simulink model "PhysicalLeanBroth"  (R2026a)
settings: Solver=VariableStepAuto  StopTime=14400
undefined symbols (not defined in the file): Fault_T_Kettle1, Fault_T_Kettle2, Fault_T_Pack, Fault_T_Prep, Fault_T_QC, LB_PackRate_bph, LB_QCRate_bph, LB_Resupply_bph, Recipe_Block_s, Recipe_Count, Resupply_Cutoff_T, Transport_Latency_s, Transport_Rate_bph
(part 1 of 2)
settings Model: DataDictionary=PhysicalLeanBrothData.sldd  Creator=sarah  LastModifiedBy=sarah

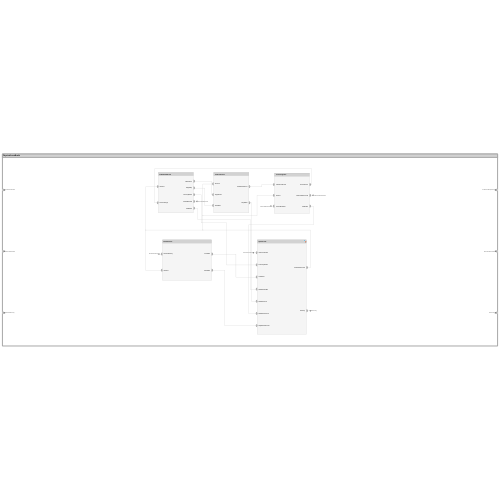
[thumbnail: Simulink's stored preview of the top-level diagram]
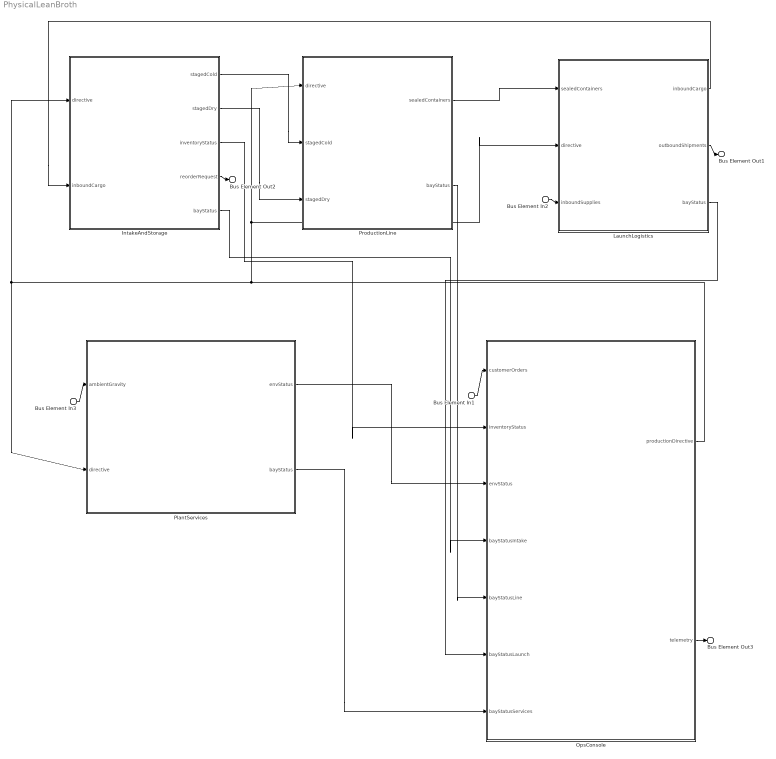
== system PhysicalLeanBroth ==
  Bus Element In1 : Inport  PortName=CustomerOrders
  Bus Element In2 : Inport  Port=2  PortName=InboundSupplies
  Bus Element In3 : Inport  Port=3  PortName=AmbientGravity
  IntakeAndStorage : Subsystem
      settings: PortSchema="{\"entries\":[{\"content\":{\"headerSize\":26,\"margin\":15,\"minimumSpacing\":25,\"sides\":[{\"content\":{\"connectorIds\":[\"In1\",\"In2\"]},\"type\":\"ConnectorPlacement.EquallySpacedRectSide\",\"uuid\":\"3a94c7fc-0b9e-4df5-a2de-1d2483378dcb\"},{\"content\":{\"connectorIds\":[\"Out1\",\"Out2\",\"Out3\",\"Out4\",\"Out5\"],\"side\":\"RIGHT\"},\"type\":\"ConnectorPlacement.EquallySpacedRectSide\",\"uuid\":\"607e1f04-41cc-4c9a-b401-96cdf33819d0\"},{\"content\":{\"side\":\"TOP\"},\"type\":\"ConnectorPlacement.EquallySpacedRectSide\",\"uuid\":\"2ee07fc7-54c6-4cee-9888-3f37ad01f332\"}]},\"type\":\"ConnectorPlacement.EquallySpacedConnector\",\"uuid\":\"f91f3af9-eaeb-4625-ae6e-5ceb7fb8b64c\"}],\"packageUris\":[\"http://schema.mathworks.com/mf0/Connector/R2020b\"],\"version\":\"1.0\"}"
  LaunchLogistics : Subsystem
      settings: PortSchema="{\"entries\":[{\"content\":{\"headerSize\":26,\"margin\":15,\"minimumSpacing\":25,\"sides\":[{\"content\":{\"connectorIds\":[\"In1\",\"In2\",\"In3\"]},\"type\":\"ConnectorPlacement.EquallySpacedRectSide\",\"uuid\":\"3a94c7fc-0b9e-4df5-a2de-1d2483378dcb\"},{\"content\":{\"connectorIds\":[\"Out1\",\"Out2\",\"Out3\"],\"side\":\"RIGHT\"},\"type\":\"ConnectorPlacement.EquallySpacedRectSide\",\"uuid\":\"607e1f04-41cc-4c9a-b401-96cdf33819d0\"},{\"content\":{\"side\":\"TOP\"},\"type\":\"ConnectorPlacement.EquallySpacedRectSide\",\"uuid\":\"2ee07fc7-54c6-4cee-9888-3f37ad01f332\"}]},\"type\":\"ConnectorPlacement.EquallySpacedConnector\",\"uuid\":\"f91f3af9-eaeb-4625-ae6e-5ceb7fb8b64c\"}],\"packageUris\":[\"http://schema.mathworks.com/mf0/Connector/R2020b\"],\"version\":\"1.0\"}"
  OpsConsole : Subsystem
      settings: PortSchema="{\"entries\":[{\"content\":{\"headerSize\":26,\"margin\":15,\"minimumSpacing\":25,\"sides\":[{\"content\":{\"connectorIds\":[\"In1\",\"In2\",\"In3\",\"In4\",\"In5\",\"In6\",\"In7\"]},\"type\":\"ConnectorPlacement.EquallySpacedRectSide\",\"uuid\":\"f830f98a-8e8b-4468-adf4-d6eab644987f\"},{\"content\":{\"connectorIds\":[\"Out1\",\"Out2\"],\"side\":\"RIGHT\"},\"type\":\"ConnectorPlacement.EquallySpacedRectSide\",\"uuid\":\"7e0d0116-b3ba-4668-b638-30d0f54ba087\"},{\"content\":{\"side\":\"TOP\"},\"type\":\"ConnectorPlacement.EquallySpacedRectSide\",\"uuid\":\"7b4146d3-46d2-45ca-8c34-b106f0d8cedd\"}]},\"type\":\"ConnectorPlacement.EquallySpacedConnector\",\"uuid\":\"3d911b2d-a78f-42ea-b869-5e09982d9f54\"}],\"packageUris\":[\"http://schema.mathworks.com/mf0/Connector/R2020b\"],\"version\":\"1.0\"}"
  PlantServices : Subsystem
      settings: PortSchema="{\"entries\":[{\"content\":{\"headerSize\":26,\"margin\":15,\"minimumSpacing\":25,\"sides\":[{\"content\":{\"connectorIds\":[\"In1\",\"In2\"]},\"type\":\"ConnectorPlacement.EquallySpacedRectSide\",\"uuid\":\"3a94c7fc-0b9e-4df5-a2de-1d2483378dcb\"},{\"content\":{\"connectorIds\":[\"Out1\",\"Out2\"],\"side\":\"RIGHT\"},\"type\":\"ConnectorPlacement.EquallySpacedRectSide\",\"uuid\":\"607e1f04-41cc-4c9a-b401-96cdf33819d0\"},{\"content\":{\"side\":\"TOP\"},\"type\":\"ConnectorPlacement.EquallySpacedRectSide\",\"uuid\":\"2ee07fc7-54c6-4cee-9888-3f37ad01f332\"}]},\"type\":\"ConnectorPlacement.EquallySpacedConnector\",\"uuid\":\"f91f3af9-eaeb-4625-ae6e-5ceb7fb8b64c\"}],\"packageUris\":[\"http://schema.mathworks.com/mf0/Connector/R2020b\"],\"version\":\"1.0\"}"
  ProductionLine : Subsystem
      settings: PortSchema="{\"entries\":[{\"content\":{\"headerSize\":26,\"margin\":15,\"minimumSpacing\":25,\"sides\":[{\"content\":{\"connectorIds\":[\"In1\",\"In2\",\"In3\"]},\"type\":\"ConnectorPlacement.EquallySpacedRectSide\",\"uuid\":\"3a94c7fc-0b9e-4df5-a2de-1d2483378dcb\"},{\"content\":{\"connectorIds\":[\"Out1\",\"Out2\"],\"side\":\"RIGHT\"},\"type\":\"ConnectorPlacement.EquallySpacedRectSide\",\"uuid\":\"607e1f04-41cc-4c9a-b401-96cdf33819d0\"},{\"content\":{\"side\":\"TOP\"},\"type\":\"ConnectorPlacement.EquallySpacedRectSide\",\"uuid\":\"2ee07fc7-54c6-4cee-9888-3f37ad01f332\"}]},\"type\":\"ConnectorPlacement.EquallySpacedConnector\",\"uuid\":\"f91f3af9-eaeb-4625-ae6e-5ceb7fb8b64c\"}],\"packageUris\":[\"http://schema.mathworks.com/mf0/Connector/R2020b\"],\"version\":\"1.0\"}"
  Bus Element Out1 : Outport  PortName=OutboundShipments
  Bus Element Out2 : Outport  Port=2  PortName=ReorderRequests
  Bus Element Out3 : Outport  Port=3  PortName=Telemetry
  wires:
  Bus Element In3/1 -> PlantServices/1(ambientGravity)
  PlantServices/1(envStatus) -> OpsConsole/3(envStatus)
  ProductionLine/2(bayStatus) -> OpsConsole/5(bayStatusLine)
  Bus Element In1/1 -> OpsConsole/1(customerOrders)
  OpsConsole/1(productionDirective) -> PlantServices/2(directive), IntakeAndStorage/1(directive), ProductionLine/1(directive), LaunchLogistics/2(directive)
  ProductionLine/1(sealedContainers) -> LaunchLogistics/1(sealedContainers)
  PlantServices/2(bayStatus) -> OpsConsole/7(bayStatusServices)
  Bus Element In2/1 -> LaunchLogistics/3(inboundSupplies)
  OpsConsole/2(telemetry) -> Bus Element Out3/1
  IntakeAndStorage/1(stagedCold) -> ProductionLine/2(stagedCold)
  LaunchLogistics/1(inboundCargo) -> IntakeAndStorage/2(inboundCargo)
  LaunchLogistics/2(outboundShipments) -> Bus Element Out1/1
  LaunchLogistics/3(bayStatus) -> OpsConsole/6(bayStatusLaunch)
  IntakeAndStorage/2(stagedDry) -> ProductionLine/3(stagedDry)
  IntakeAndStorage/3(inventoryStatus) -> OpsConsole/2(inventoryStatus)
  IntakeAndStorage/4(reorderRequest) -> Bus Element Out2/1
  IntakeAndStorage/5(bayStatus) -> OpsConsole/4(bayStatusIntake)

== system PhysicalLeanBroth/IntakeAndStorage ==
  Bus Element In1 : Inport  PortName=directive
  Bus Element In2 : Inport  Port=2  PortName=inboundCargo
  BarcodeInventorySystem : Subsystem
      settings: PortSchema="{\"entries\":[{\"content\":{\"headerSize\":26,\"margin\":15,\"minimumSpacing\":25,\"sides\":[{\"content\":{\"connectorIds\":[\"In1\",\"In2\"]},\"type\":\"ConnectorPlacement.EquallySpacedRectSide\",\"uuid\":\"f830f98a-8e8b-4468-adf4-d6eab644987f\"},{\"content\":{\"connectorIds\":[\"Out1\",\"Out2\"],\"side\":\"RIGHT\"},\"type\":\"ConnectorPlacement.EquallySpacedRectSide\",\"uuid\":\"7e0d0116-b3ba-4668-b638-30d0f54ba087\"},{\"content\":{\"side\":\"TOP\"},\"type\":\"ConnectorPlacement.EquallySpacedRectSide\",\"uuid\":\"7b4146d3-46d2-45ca-8c34-b106f0d8cedd\"}]},\"type\":\"ConnectorPlacement.EquallySpacedConnector\",\"uuid\":\"3d911b2d-a78f-42ea-b869-5e09982d9f54\"}],\"packageUris\":[\"http://schema.mathworks.com/mf0/Connector/R2020b\"],\"version\":\"1.0\"}"
  ColdStoreLocker : Subsystem
      settings: PortSchema="{\"entries\":[{\"content\":{\"headerSize\":26,\"margin\":15,\"minimumSpacing\":25,\"sides\":[{\"content\":{\"connectorIds\":[\"In1\",\"In2\"]},\"type\":\"ConnectorPlacement.EquallySpacedRectSide\",\"uuid\":\"f830f98a-8e8b-4468-adf4-d6eab644987f\"},{\"content\":{\"connectorIds\":[\"Out1\",\"Out2\",\"Out3\"],\"side\":\"RIGHT\"},\"type\":\"ConnectorPlacement.EquallySpacedRectSide\",\"uuid\":\"7e0d0116-b3ba-4668-b638-30d0f54ba087\"},{\"content\":{\"side\":\"TOP\"},\"type\":\"ConnectorPlacement.EquallySpacedRectSide\",\"uuid\":\"7b4146d3-46d2-45ca-8c34-b106f0d8cedd\"}]},\"type\":\"ConnectorPlacement.EquallySpacedConnector\",\"uuid\":\"3d911b2d-a78f-42ea-b869-5e09982d9f54\"}],\"packageUris\":[\"http://schema.mathworks.com/mf0/Connector/R2020b\"],\"version\":\"1.0\"}"
  DryGoodsRack : Subsystem
      settings: PortSchema="{\"entries\":[{\"content\":{\"headerSize\":26,\"margin\":15,\"minimumSpacing\":25,\"sides\":[{\"content\":{\"connectorIds\":[\"In1\",\"In2\"]},\"type\":\"ConnectorPlacement.EquallySpacedRectSide\",\"uuid\":\"f830f98a-8e8b-4468-adf4-d6eab644987f\"},{\"content\":{\"connectorIds\":[\"Out1\",\"Out2\",\"Out3\"],\"side\":\"RIGHT\"},\"type\":\"ConnectorPlacement.EquallySpacedRectSide\",\"uuid\":\"7e0d0116-b3ba-4668-b638-30d0f54ba087\"},{\"content\":{\"side\":\"TOP\"},\"type\":\"ConnectorPlacement.EquallySpacedRectSide\",\"uuid\":\"7b4146d3-46d2-45ca-8c34-b106f0d8cedd\"}]},\"type\":\"ConnectorPlacement.EquallySpacedConnector\",\"uuid\":\"3d911b2d-a78f-42ea-b869-5e09982d9f54\"}],\"packageUris\":[\"http://schema.mathworks.com/mf0/Connector/R2020b\"],\"version\":\"1.0\"}"
  IntakeController : Subsystem
      settings: PortSchema="{\"entries\":[{\"content\":{\"headerSize\":26,\"margin\":15,\"minimumSpacing\":25,\"sides\":[{\"content\":{\"connectorIds\":[\"In1\",\"In2\",\"In3\",\"In4\"]},\"type\":\"ConnectorPlacement.EquallySpacedRectSide\",\"uuid\":\"0731d988-4a26-4db6-8347-b78d2aa6954f\"},{\"content\":{\"connectorIds\":[\"Out1\",\"Out2\"],\"side\":\"RIGHT\"},\"type\":\"ConnectorPlacement.EquallySpacedRectSide\",\"uuid\":\"6e8ac7ed-a816-4c7e-8f31-c61224c9ac03\"},{\"content\":{\"side\":\"TOP\"},\"type\":\"ConnectorPlacement.EquallySpacedRectSide\",\"uuid\":\"7c48a918-2743-4697-bc21-ce4fb8bbcea2\"}]},\"type\":\"ConnectorPlacement.EquallySpacedConnector\",\"uuid\":\"5e30be34-c1af-4919-9af8-d4df8145ecd1\"}],\"packageUris\":[\"http://schema.mathworks.com/mf0/Connector/R2020b\"],\"version\":\"1.0\"}"
  ManualReceivingBay : Subsystem
      settings: PortSchema="{\"entries\":[{\"content\":{\"headerSize\":26,\"margin\":15,\"minimumSpacing\":25,\"sides\":[{\"content\":{\"connectorIds\":[\"In1\",\"In2\"]},\"type\":\"ConnectorPlacement.EquallySpacedRectSide\",\"uuid\":\"f830f98a-8e8b-4468-adf4-d6eab644987f\"},{\"content\":{\"connectorIds\":[\"Out1\",\"Out2\"],\"side\":\"RIGHT\"},\"type\":\"ConnectorPlacement.EquallySpacedRectSide\",\"uuid\":\"7e0d0116-b3ba-4668-b638-30d0f54ba087\"},{\"content\":{\"side\":\"TOP\"},\"type\":\"ConnectorPlacement.EquallySpacedRectSide\",\"uuid\":\"7b4146d3-46d2-45ca-8c34-b106f0d8cedd\"}]},\"type\":\"ConnectorPlacement.EquallySpacedConnector\",\"uuid\":\"3d911b2d-a78f-42ea-b869-5e09982d9f54\"}],\"packageUris\":[\"http://schema.mathworks.com/mf0/Connector/R2020b\"],\"version\":\"1.0\"}"
  Bus Element Out1 : Outport  PortName=stagedCold
  Bus Element Out2 : Outport  Port=2  PortName=stagedDry
  Bus Element Out3 : Outport  Port=3  PortName=inventoryStatus
  Bus Element Out7 : Outport  Port=4  PortName=reorderRequest
  Bus Element Out8 : Outport  Port=5  PortName=bayStatus
  wires:
  ManualReceivingBay/1(receivedIngredients) -> DryGoodsRack/1(receivedIngredients), ColdStoreLocker/1(receivedIngredients)
  Bus Element In2/1 -> ManualReceivingBay/1(inboundCargo)
  Bus Element In1/1 -> IntakeController/1(directive)
  ColdStoreLocker/2(stockCold) -> BarcodeInventorySystem/1(stockCold)
  DryGoodsRack/2(stockDry) -> BarcodeInventorySystem/2(stockDry)
  IntakeController/1(bayDirective) -> ManualReceivingBay/2(directive), ColdStoreLocker/2(directive), DryGoodsRack/2(directive)
  ManualReceivingBay/2(statusReceive) -> IntakeController/4(statusReceive)
  IntakeController/2(bayStatus) -> Bus Element Out8/1
  DryGoodsRack/1(stagedDry) -> Bus Element Out2/1
  ColdStoreLocker/1(stagedCold) -> Bus Element Out1/1
  DryGoodsRack/3(statusDryStore) -> IntakeController/3(statusDryStore)
  ColdStoreLocker/3(statusColdStore) -> IntakeController/2(statusColdStore)
  BarcodeInventorySystem/1(inventoryStatus) -> Bus Element Out3/1
  BarcodeInventorySystem/2(reorderRequest) -> Bus Element Out7/1

== system PhysicalLeanBroth/LaunchLogistics ==
  Bus Element In2 : Inport  PortName=sealedContainers
  Bus Element In3 : Inport  Port=2  PortName=directive
  Bus Element In5 : Inport  Port=3  PortName=inboundSupplies
  LaunchController : Subsystem
      settings: PortSchema="{\"entries\":[{\"content\":{\"headerSize\":26,\"margin\":15,\"minimumSpacing\":25,\"sides\":[{\"content\":{\"connectorIds\":[\"In1\",\"In2\",\"In3\",\"In4\"]},\"type\":\"ConnectorPlacement.EquallySpacedRectSide\",\"uuid\":\"0731d988-4a26-4db6-8347-b78d2aa6954f\"},{\"content\":{\"connectorIds\":[\"Out1\",\"Out2\"],\"side\":\"RIGHT\"},\"type\":\"ConnectorPlacement.EquallySpacedRectSide\",\"uuid\":\"6e8ac7ed-a816-4c7e-8f31-c61224c9ac03\"},{\"content\":{\"side\":\"TOP\"},\"type\":\"ConnectorPlacement.EquallySpacedRectSide\",\"uuid\":\"7c48a918-2743-4697-bc21-ce4fb8bbcea2\"}]},\"type\":\"ConnectorPlacement.EquallySpacedConnector\",\"uuid\":\"5e30be34-c1af-4919-9af8-d4df8145ecd1\"}],\"packageUris\":[\"http://schema.mathworks.com/mf0/Connector/R2020b\"],\"version\":\"1.0\"}"
  RefuelSkid : Subsystem
      settings: PortSchema="{\"entries\":[{\"content\":{\"headerSize\":26,\"margin\":15,\"minimumSpacing\":25,\"sides\":[{\"content\":{\"connectorIds\":[\"In1\"]},\"type\":\"ConnectorPlacement.EquallySpacedRectSide\",\"uuid\":\"f830f98a-8e8b-4468-adf4-d6eab644987f\"},{\"content\":{\"connectorIds\":[\"Out1\"],\"side\":\"RIGHT\"},\"type\":\"ConnectorPlacement.EquallySpacedRectSide\",\"uuid\":\"7e0d0116-b3ba-4668-b638-30d0f54ba087\"},{\"content\":{\"side\":\"TOP\"},\"type\":\"ConnectorPlacement.EquallySpacedRectSide\",\"uuid\":\"7b4146d3-46d2-45ca-8c34-b106f0d8cedd\"}]},\"type\":\"ConnectorPlacement.EquallySpacedConnector\",\"uuid\":\"3d911b2d-a78f-42ea-b869-5e09982d9f54\"}],\"packageUris\":[\"http://schema.mathworks.com/mf0/Connector/R2020b\"],\"version\":\"1.0\"}"
  SharedCraneDock : Subsystem
      settings: PortSchema="{\"entries\":[{\"content\":{\"headerSize\":26,\"margin\":15,\"minimumSpacing\":25,\"sides\":[{\"content\":{\"connectorIds\":[\"In1\",\"In2\"]},\"type\":\"ConnectorPlacement.EquallySpacedRectSide\",\"uuid\":\"f830f98a-8e8b-4468-adf4-d6eab644987f\"},{\"content\":{\"connectorIds\":[\"Out1\",\"Out2\",\"Out3\"],\"side\":\"RIGHT\"},\"type\":\"ConnectorPlacement.EquallySpacedRectSide\",\"uuid\":\"7e0d0116-b3ba-4668-b638-30d0f54ba087\"},{\"content\":{\"side\":\"TOP\"},\"type\":\"ConnectorPlacement.EquallySpacedRectSide\",\"uuid\":\"7b4146d3-46d2-45ca-8c34-b106f0d8cedd\"}]},\"type\":\"ConnectorPlacement.EquallySpacedConnector\",\"uuid\":\"3d911b2d-a78f-42ea-b869-5e09982d9f54\"}],\"packageUris\":[\"http://schema.mathworks.com/mf0/Connector/R2020b\"],\"version\":\"1.0\"}"
  TriPadLandingField : Subsystem
      settings: PortSchema="{\"entries\":[{\"content\":{\"headerSize\":26,\"margin\":15,\"minimumSpacing\":25,\"sides\":[{\"content\":{\"connectorIds\":[\"In1\",\"In2\",\"In3\",\"In4\"]},\"type\":\"ConnectorPlacement.EquallySpacedRectSide\",\"uuid\":\"f830f98a-8e8b-4468-adf4-d6eab644987f\"},{\"content\":{\"connectorIds\":[\"Out1\",\"Out2\",\"Out3\"],\"side\":\"RIGHT\"},\"type\":\"ConnectorPlacement.EquallySpacedRectSide\",\"uuid\":\"7e0d0116-b3ba-4668-b638-30d0f54ba087\"},{\"content\":{\"side\":\"TOP\"},\"type\":\"ConnectorPlacement.EquallySpacedRectSide\",\"uuid\":\"7b4146d3-46d2-45ca-8c34-b106f0d8cedd\"}]},\"type\":\"ConnectorPlacement.EquallySpacedConnector\",\"uuid\":\"3d911b2d-a78f-42ea-b869-5e09982d9f54\"}],\"packageUris\":[\"http://schema.mathworks.com/mf0/Connector/R2020b\"],\"version\":\"1.0\"}"
  Bus Element Out3 : Outport  PortName=inboundCargo
  Bus Element Out5 : Outport  Port=2  PortName=outboundShipments
  Bus Element Out6 : Outport  Port=3  PortName=bayStatus
  wires:
  TriPadLandingField/3(statusFleet) -> LaunchController/4(statusFleet)
  TriPadLandingField/1(inboundCargo) -> Bus Element Out3/1
  Bus Element In2/1 -> SharedCraneDock/1(sealedContainers)
  Bus Element In5/1 -> TriPadLandingField/4(inboundSupplies)
  TriPadLandingField/2(outboundShipments) -> Bus Element Out5/1
  SharedCraneDock/3(statusDispatch) -> LaunchController/3(statusDispatch)
  SharedCraneDock/1(loadedShipment) -> TriPadLandingField/1(loadedShipment)
  RefuelSkid/1(statusRefuel) -> LaunchController/2(statusRefuel)
  SharedCraneDock/2(manifest) -> TriPadLandingField/2(manifest)
  Bus Element In3/1 -> LaunchController/1(directive)
  LaunchController/1(bayDirective) -> RefuelSkid/1(directive), SharedCraneDock/2(directive), TriPadLandingField/3(directive)
  LaunchController/2(bayStatus) -> Bus Element Out6/1

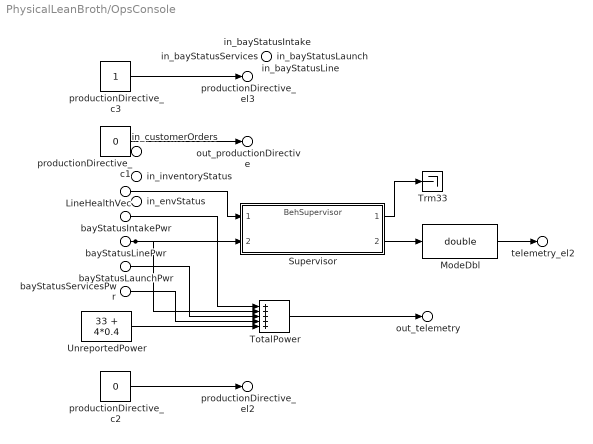
== system PhysicalLeanBroth/OpsConsole ==
  in_customerOrders : Inport  PortName=customerOrders
  in_inventoryStatus : Inport  Port=2  PortName=inventoryStatus
  in_envStatus : Inport  Port=3  PortName=envStatus
  in_bayStatusIntake : Inport  Port=4  PortName=bayStatusIntake
  bayStatusIntakePwr : Inport  Port=4  PortName=bayStatusIntake  Element=power_kW
  in_bayStatusLine : Inport  Port=5  PortName=bayStatusLine  Element=power_kW
  bayStatusLinePwr : Inport  Port=5  PortName=bayStatusLine  Element=power_kW
  LineHealthVec : Inport  Port=5  PortName=bayStatusLine  Element=lineHealth
  in_bayStatusLaunch : Inport  Port=6  PortName=bayStatusLaunch
  bayStatusLaunchPwr : Inport  Port=6  PortName=bayStatusLaunch  Element=power_kW
  in_bayStatusServices : Inport  Port=7  PortName=bayStatusServices
  bayStatusServicesPwr : Inport  Port=7  PortName=bayStatusServices  Element=power_kW
  ModeDbl : DataTypeConversion  OutDataTypeStr=double  SaturateOnIntegerOverflow=off  RndMeth=Floor
  Supervisor : ModelReference  ModelNameDialog=BehSupervisor  ParameterArgumentNames=NumLines  ParameterArgumentValues=LB_NumLines  UsingDefaultArgumentValue=0  SimulationMode=Normal  ModelReferenceVersion=1.7
  TotalPower : Sum  Inputs=+++++
  Trm33 : Terminator
  UnreportedPower : Constant  Value=33 + 4*0.4
  productionDirective_c1 : Constant  Value=0
  productionDirective_c2 : Constant  Value=0
  productionDirective_c3 : Constant
  out_productionDirective : Outport  PortName=productionDirective  Element=cmdType
  productionDirective_el2 : Outport  PortName=productionDirective  Element=targetId
  productionDirective_el3 : Outport  PortName=productionDirective  Element=setpoint
  out_telemetry : Outport  Port=2  PortName=telemetry  Element=totalPower_kW
  telemetry_el2 : Outport  Port=2  PortName=telemetry  Element=plantMode
  wires:
  UnreportedPower/1 -> TotalPower/5
  productionDirective_c3/1 -> productionDirective_el3/1
  productionDirective_c1/1 -> out_productionDirective/1
  bayStatusServicesPwr/1 -> TotalPower/4
  bayStatusLaunchPwr/1 -> TotalPower/3
  LineHealthVec/1 -> Supervisor/1
  productionDirective_c2/1 -> productionDirective_el2/1
  bayStatusLinePwr/1 -> Supervisor/2, TotalPower/2
  bayStatusIntakePwr/1 -> TotalPower/1
  Supervisor/1 -> Trm33/1
  Supervisor/2 -> ModeDbl/1
  TotalPower/1 -> out_telemetry/1
  ModeDbl/1 -> telemetry_el2/1

== system PhysicalLeanBroth/PlantServices ==
  Bus Element In1 : Inport  PortName=ambientGravity
  Bus Element In2 : Inport  Port=2  PortName=directive
  Bus Element In4 : Inport  Port=2  PortName=directive
  AGVCartPool : Subsystem
      settings: PortSchema="{\"entries\":[{\"content\":{\"headerSize\":26,\"margin\":15,\"minimumSpacing\":25,\"sides\":[{\"content\":{\"connectorIds\":[\"In1\"]},\"type\":\"ConnectorPlacement.EquallySpacedRectSide\",\"uuid\":\"f830f98a-8e8b-4468-adf4-d6eab644987f\"},{\"content\":{\"connectorIds\":[\"Out1\"],\"side\":\"RIGHT\"},\"type\":\"ConnectorPlacement.EquallySpacedRectSide\",\"uuid\":\"7e0d0116-b3ba-4668-b638-30d0f54ba087\"},{\"content\":{\"side\":\"TOP\"},\"type\":\"ConnectorPlacement.EquallySpacedRectSide\",\"uuid\":\"7b4146d3-46d2-45ca-8c34-b106f0d8cedd\"}]},\"type\":\"ConnectorPlacement.EquallySpacedConnector\",\"uuid\":\"3d911b2d-a78f-42ea-b869-5e09982d9f54\"}],\"packageUris\":[\"http://schema.mathworks.com/mf0/Connector/R2020b\"],\"version\":\"1.0\"}"
  CompactFissionReactor : Subsystem
      settings: PortSchema="{\"entries\":[{\"content\":{\"headerSize\":26,\"margin\":15,\"minimumSpacing\":25,\"sides\":[{\"content\":{\"connectorIds\":[\"In1\"]},\"type\":\"ConnectorPlacement.EquallySpacedRectSide\",\"uuid\":\"f830f98a-8e8b-4468-adf4-d6eab644987f\"},{\"content\":{\"connectorIds\":[\"Out1\"],\"side\":\"RIGHT\"},\"type\":\"ConnectorPlacement.EquallySpacedRectSide\",\"uuid\":\"7e0d0116-b3ba-4668-b638-30d0f54ba087\"},{\"content\":{\"side\":\"TOP\"},\"type\":\"ConnectorPlacement.EquallySpacedRectSide\",\"uuid\":\"7b4146d3-46d2-45ca-8c34-b106f0d8cedd\"}]},\"type\":\"ConnectorPlacement.EquallySpacedConnector\",\"uuid\":\"3d911b2d-a78f-42ea-b869-5e09982d9f54\"}],\"packageUris\":[\"http://schema.mathworks.com/mf0/Connector/R2020b\"],\"version\":\"1.0\"}"
  GravityCompUnit : Subsystem
      settings: PortSchema="{\"entries\":[{\"content\":{\"headerSize\":26,\"margin\":15,\"minimumSpacing\":25,\"sides\":[{\"content\":{\"connectorIds\":[\"In1\"]},\"type\":\"ConnectorPlacement.EquallySpacedRectSide\",\"uuid\":\"f830f98a-8e8b-4468-adf4-d6eab644987f\"},{\"content\":{\"connectorIds\":[\"Out1\"],\"side\":\"RIGHT\"},\"type\":\"ConnectorPlacement.EquallySpacedRectSide\",\"uuid\":\"7e0d0116-b3ba-4668-b638-30d0f54ba087\"},{\"content\":{\"side\":\"TOP\"},\"type\":\"ConnectorPlacement.EquallySpacedRectSide\",\"uuid\":\"7b4146d3-46d2-45ca-8c34-b106f0d8cedd\"}]},\"type\":\"ConnectorPlacement.EquallySpacedConnector\",\"uuid\":\"3d911b2d-a78f-42ea-b869-5e09982d9f54\"}],\"packageUris\":[\"http://schema.mathworks.com/mf0/Connector/R2020b\"],\"version\":\"1.0\"}"
  ServicesController : Subsystem
      settings: PortSchema="{\"entries\":[{\"content\":{\"headerSize\":26,\"margin\":15,\"minimumSpacing\":25,\"sides\":[{\"content\":{\"connectorIds\":[\"In1\",\"In2\",\"In3\"]},\"type\":\"ConnectorPlacement.EquallySpacedRectSide\",\"uuid\":\"0731d988-4a26-4db6-8347-b78d2aa6954f\"},{\"content\":{\"connectorIds\":[\"Out1\",\"Out2\"],\"side\":\"RIGHT\"},\"type\":\"ConnectorPlacement.EquallySpacedRectSide\",\"uuid\":\"6e8ac7ed-a816-4c7e-8f31-c61224c9ac03\"},{\"content\":{\"side\":\"TOP\"},\"type\":\"ConnectorPlacement.EquallySpacedRectSide\",\"uuid\":\"7c48a918-2743-4697-bc21-ce4fb8bbcea2\"}]},\"type\":\"ConnectorPlacement.EquallySpacedConnector\",\"uuid\":\"5e30be34-c1af-4919-9af8-d4df8145ecd1\"}],\"packageUris\":[\"http://schema.mathworks.com/mf0/Connector/R2020b\"],\"version\":\"1.0\"}"
  Bus Element Out1 : Outport  PortName=envStatus
  Bus Element Out4 : Outport  Port=2  PortName=bayStatus
  wires:
  Bus Element In1/1 -> GravityCompUnit/1(ambientGravity)
  Bus Element In4/1 -> AGVCartPool/1(transportDirective)
  ServicesController/2(bayStatus) -> Bus Element Out4/1
  AGVCartPool/1(statusTransport) -> ServicesController/2(statusTransport)
  GravityCompUnit/1(envStatus) -> Bus Element Out1/1
  ServicesController/1(bayDirective) -> CompactFissionReactor/1(directive)
  Bus Element In2/1 -> ServicesController/1(directive)
  CompactFissionReactor/1(statusPower) -> ServicesController/3(statusPower)

== system PhysicalLeanBroth/ProductionLine ==
  Bus Element In1 : Inport  PortName=directive
  Bus Element In4 : Inport  Port=2  PortName=stagedCold
  Bus Element In5 : Inport  Port=3  PortName=stagedDry
  BatchKettle1 : Subsystem
      settings: PortSchema="{\"entries\":[{\"content\":{\"headerSize\":26,\"margin\":15,\"minimumSpacing\":25,\"sides\":[{\"content\":{\"connectorIds\":[\"In1\",\"In2\"]},\"type\":\"ConnectorPlacement.EquallySpacedRectSide\",\"uuid\":\"f830f98a-8e8b-4468-adf4-d6eab644987f\"},{\"content\":{\"connectorIds\":[\"Out1\",\"Out2\"],\"side\":\"RIGHT\"},\"type\":\"ConnectorPlacement.EquallySpacedRectSide\",\"uuid\":\"7e0d0116-b3ba-4668-b638-30d0f54ba087\"},{\"content\":{\"side\":\"TOP\"},\"type\":\"ConnectorPlacement.EquallySpacedRectSide\",\"uuid\":\"7b4146d3-46d2-45ca-8c34-b106f0d8cedd\"}]},\"type\":\"ConnectorPlacement.EquallySpacedConnector\",\"uuid\":\"3d911b2d-a78f-42ea-b869-5e09982d9f54\"}],\"packageUris\":[\"http://schema.mathworks.com/mf0/Connector/R2020b\"],\"version\":\"1.0\"}"
  BatchKettle2 : Subsystem
      settings: PortSchema="{\"entries\":[{\"content\":{\"headerSize\":26,\"margin\":15,\"minimumSpacing\":25,\"sides\":[{\"content\":{\"connectorIds\":[\"In1\",\"In2\"]},\"type\":\"ConnectorPlacement.EquallySpacedRectSide\",\"uuid\":\"f830f98a-8e8b-4468-adf4-d6eab644987f\"},{\"content\":{\"connectorIds\":[\"Out1\",\"Out2\"],\"side\":\"RIGHT\"},\"type\":\"ConnectorPlacement.EquallySpacedRectSide\",\"uuid\":\"7e0d0116-b3ba-4668-b638-30d0f54ba087\"},{\"content\":{\"side\":\"TOP\"},\"type\":\"ConnectorPlacement.EquallySpacedRectSide\",\"uuid\":\"7b4146d3-46d2-45ca-8c34-b106f0d8cedd\"}]},\"type\":\"ConnectorPlacement.EquallySpacedConnector\",\"uuid\":\"3d911b2d-a78f-42ea-b869-5e09982d9f54\"}],\"packageUris\":[\"http://schema.mathworks.com/mf0/Connector/R2020b\"],\"version\":\"1.0\"}"
  LineController : Subsystem
      settings: PortSchema="{\"entries\":[{\"content\":{\"headerSize\":26,\"margin\":15,\"minimumSpacing\":25,\"sides\":[{\"content\":{\"connectorIds\":[\"In1\",\"In2\",\"In3\",\"In4\",\"In5\",\"In6\"]},\"type\":\"ConnectorPlacement.EquallySpacedRectSide\",\"uuid\":\"0731d988-4a26-4db6-8347-b78d2aa6954f\"},{\"content\":{\"connectorIds\":[\"Out1\",\"Out2\"],\"side\":\"RIGHT\"},\"type\":\"ConnectorPlacement.EquallySpacedRectSide\",\"uuid\":\"6e8ac7ed-a816-4c7e-8f31-c61224c9ac03\"},{\"content\":{\"side\":\"TOP\"},\"type\":\"ConnectorPlacement.EquallySpacedRectSide\",\"uuid\":\"7c48a918-2743-4697-bc21-ce4fb8bbcea2\"}]},\"type\":\"ConnectorPlacement.EquallySpacedConnector\",\"uuid\":\"5e30be34-c1af-4919-9af8-d4df8145ecd1\"}],\"packageUris\":[\"http://schema.mathworks.com/mf0/Connector/R2020b\"],\"version\":\"1.0\"}"
  PrepWorkstation : Subsystem
      settings: PortSchema="{\"entries\":[{\"content\":{\"headerSize\":26,\"margin\":15,\"minimumSpacing\":25,\"sides\":[{\"content\":{\"connectorIds\":[\"In1\",\"In2\",\"In3\"]},\"type\":\"ConnectorPlacement.EquallySpacedRectSide\",\"uuid\":\"f830f98a-8e8b-4468-adf4-d6eab644987f\"},{\"content\":{\"connectorIds\":[\"Out1\",\"Out2\"],\"side\":\"RIGHT\"},\"type\":\"ConnectorPlacement.EquallySpacedRectSide\",\"uuid\":\"7e0d0116-b3ba-4668-b638-30d0f54ba087\"},{\"content\":{\"side\":\"TOP\"},\"type\":\"ConnectorPlacement.EquallySpacedRectSide\",\"uuid\":\"7b4146d3-46d2-45ca-8c34-b106f0d8cedd\"}]},\"type\":\"ConnectorPlacement.EquallySpacedConnector\",\"uuid\":\"3d911b2d-a78f-42ea-b869-5e09982d9f54\"}],\"packageUris\":[\"http://schema.mathworks.com/mf0/Connector/R2020b\"],\"version\":\"1.0\"}"
  QCBench : Subsystem
      settings: PortSchema="{\"entries\":[{\"content\":{\"headerSize\":26,\"margin\":15,\"minimumSpacing\":25,\"sides\":[{\"content\":{\"connectorIds\":[\"In1\",\"In2\",\"In3\"]},\"type\":\"ConnectorPlacement.EquallySpacedRectSide\",\"uuid\":\"f830f98a-8e8b-4468-adf4-d6eab644987f\"},{\"content\":{\"connectorIds\":[\"Out1\",\"Out2\"],\"side\":\"RIGHT\"},\"type\":\"ConnectorPlacement.EquallySpacedRectSide\",\"uuid\":\"7e0d0116-b3ba-4668-b638-30d0f54ba087\"},{\"content\":{\"side\":\"TOP\"},\"type\":\"ConnectorPlacement.EquallySpacedRectSide\",\"uuid\":\"7b4146d3-46d2-45ca-8c34-b106f0d8cedd\"}]},\"type\":\"ConnectorPlacement.EquallySpacedConnector\",\"uuid\":\"3d911b2d-a78f-42ea-b869-5e09982d9f54\"}],\"packageUris\":[\"http://schema.mathworks.com/mf0/Connector/R2020b\"],\"version\":\"1.0\"}"
  SemiAutoPackager : Subsystem
      settings: PortSchema="{\"entries\":[{\"content\":{\"headerSize\":26,\"margin\":15,\"minimumSpacing\":25,\"sides\":[{\"content\":{\"connectorIds\":[\"In1\",\"In2\"]},\"type\":\"ConnectorPlacement.EquallySpacedRectSide\",\"uuid\":\"f830f98a-8e8b-4468-adf4-d6eab644987f\"},{\"content\":{\"connectorIds\":[\"Out1\",\"Out2\"],\"side\":\"RIGHT\"},\"type\":\"ConnectorPlacement.EquallySpacedRectSide\",\"uuid\":\"7e0d0116-b3ba-4668-b638-30d0f54ba087\"},{\"content\":{\"side\":\"TOP\"},\"type\":\"ConnectorPlacement.EquallySpacedRectSide\",\"uuid\":\"7b4146d3-46d2-45ca-8c34-b106f0d8cedd\"}]},\"type\":\"ConnectorPlacement.EquallySpacedConnector\",\"uuid\":\"3d911b2d-a78f-42ea-b869-5e09982d9f54\"}],\"packageUris\":[\"http://schema.mathworks.com/mf0/Connector/R2020b\"],\"version\":\"1.0\"}"
  Bus Element Out1 : Outport  PortName=sealedContainers
  Bus Element Out7 : Outport  Port=2  PortName=bayStatus
  wires:
  Bus Element In1/1 -> LineController/1(directive)
  Bus Element In5/1 -> PrepWorkstation/2(stagedDry)
  Bus Element In4/1 -> PrepWorkstation/1(stagedCold)
  SemiAutoPackager/1(sealedContainers) -> Bus Element Out1/1
  SemiAutoPackager/2(statusPack) -> LineController/6(statusPack)
  LineController/2(bayStatus) -> Bus Element Out7/1
  PrepWorkstation/1(preppedBatch) -> BatchKettle2/1(preppedBatch), BatchKettle1/1(preppedBatch)
  PrepWorkstation/2(statusPrep) -> LineController/4(statusPrep)
  QCBench/1(approvedSoup) -> SemiAutoPackager/1(approvedSoup)
  QCBench/2(statusQA) -> LineController/5(statusQA)
  LineController/1(bayDirective) -> SemiAutoPackager/2(directive), QCBench/3(directive), BatchKettle2/2(directive), PrepWorkstation/3(directive), BatchKettle1/2(directive)
  BatchKettle1/1(cookedSoup1) -> QCBench/1(cookedSoup1)
  BatchKettle1/2(statusCook1) -> LineController/2(statusCook1)
  BatchKettle2/1(cookedSoup2) -> QCBench/2(cookedSoup2)
  BatchKettle2/2(statusCook2) -> LineController/3(statusCook2)

== system PhysicalLeanBroth/IntakeAndStorage/BarcodeInventorySystem ==
  in_stockCold : Inport  PortName=stockCold
  in_stockDry : Inport  Port=2  PortName=stockDry
  inventoryStatus_c1 : Constant
  inventoryStatus_c2 : Constant  Value=500
  inventoryStatus_c3 : Constant  Value=0
  reorderRequest_c1 : Constant
  reorderRequest_c2 : Constant  Value=0
  reorderRequest_c3 : Constant  Value=0
  out_inventoryStatus : Outport  PortName=inventoryStatus  Element=itemId
  inventoryStatus_el2 : Outport  PortName=inventoryStatus  Element=qty_units
  inventoryStatus_el3 : Outport  PortName=inventoryStatus  Element=error_pct
  out_reorderRequest : Outport  Port=2  PortName=reorderRequest  Element=itemId
  reorderRequest_el2 : Outport  Port=2  PortName=reorderRequest  Element=qty_units
  reorderRequest_el3 : Outport  Port=2  PortName=reorderRequest  Element=error_pct
  wires:
  reorderRequest_c2/1 -> reorderRequest_el2/1
  reorderRequest_c3/1 -> reorderRequest_el3/1
  reorderRequest_c1/1 -> out_reorderRequest/1
  inventoryStatus_c1/1 -> out_inventoryStatus/1
  inventoryStatus_c3/1 -> inventoryStatus_el3/1
  inventoryStatus_c2/1 -> inventoryStatus_el2/1

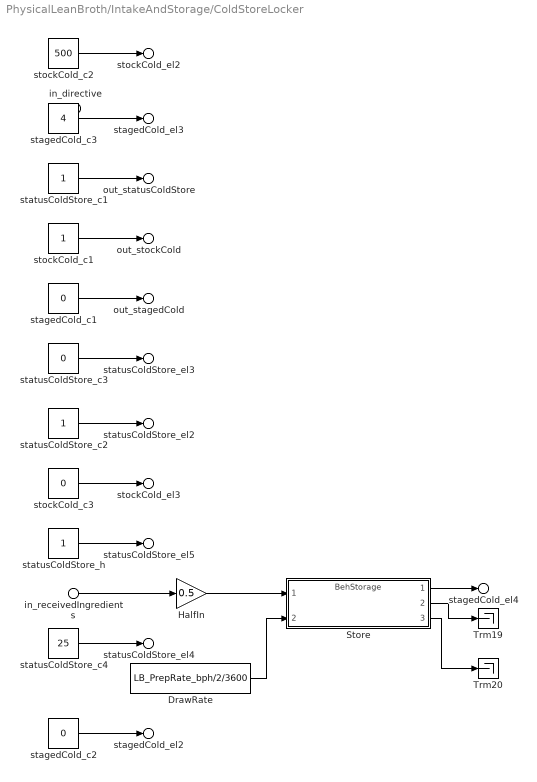
== system PhysicalLeanBroth/IntakeAndStorage/ColdStoreLocker ==
  in_receivedIngredients : Inport  PortName=receivedIngredients  Element=flow_bps
  in_directive : Inport  Port=2  PortName=directive  Element=setpoint
  DrawRate : Constant  Value=LB_PrepRate_bph/2/3600
  HalfIn : Gain  Gain=0.5
  Store : ModelReference  ModelNameDialog=BehStorage  UsingDefaultArgumentValue=0,0  SimulationMode=Normal  ModelReferenceVersion=1.4
  Trm19 : Terminator
  Trm20 : Terminator
  stagedCold_c1 : Constant  Value=0
  stagedCold_c2 : Constant  Value=0
  stagedCold_c3 : Constant  Value=4
  statusColdStore_c1 : Constant
  statusColdStore_c2 : Constant
  statusColdStore_c3 : Constant  Value=0
  statusColdStore_c4 : Constant  Value=25
  statusColdStore_h : Constant
  stockCold_c1 : Constant
  stockCold_c2 : Constant  Value=500
  stockCold_c3 : Constant  Value=0
  out_stagedCold : Outport  PortName=stagedCold  Element=palletId
  stagedCold_el2 : Outport  PortName=stagedCold  Element=mass_kg
  stagedCold_el3 : Outport  PortName=stagedCold  Element=temp_C
  stagedCold_el4 : Outport  PortName=stagedCold  Element=flow_bps
  out_stockCold : Outport  Port=2  PortName=stockCold  Element=itemId
  stockCold_el2 : Outport  Port=2  PortName=stockCold  Element=qty_units
  stockCold_el3 : Outport  Port=2  PortName=stockCold  Element=error_pct
  out_statusColdStore : Outport  Port=3  PortName=statusColdStore  Element=unitId
  statusColdStore_el2 : Outport  Port=3  PortName=statusColdStore  Element=opState
  statusColdStore_el3 : Outport  Port=3  PortName=statusColdStore  Element=faultCode
  statusColdStore_el4 : Outport  Port=3  PortName=statusColdStore  Element=power_kW
  statusColdStore_el5 : Outport  Port=3  PortName=statusColdStore  Element=health
  wires:
  stockCold_c2/1 -> stockCold_el2/1
  statusColdStore_c1/1 -> out_statusColdStore/1
  stagedCold_c3/1 -> stagedCold_el3/1
  stagedCold_c1/1 -> out_stagedCold/1
  stockCold_c1/1 -> out_stockCold/1
  statusColdStore_c3/1 -> statusColdStore_el3/1
  stockCold_c3/1 -> stockCold_el3/1
  Store/3 -> Trm20/1
  statusColdStore_c2/1 -> statusColdStore_el2/1
  statusColdStore_h/1 -> statusColdStore_el5/1
  in_receivedIngredients/1 -> HalfIn/1
  statusColdStore_c4/1 -> statusColdStore_el4/1
  stagedCold_c2/1 -> stagedCold_el2/1
  HalfIn/1 -> Store/1
  DrawRate/1 -> Store/2
  Store/1 -> stagedCold_el4/1
  Store/2 -> Trm19/1

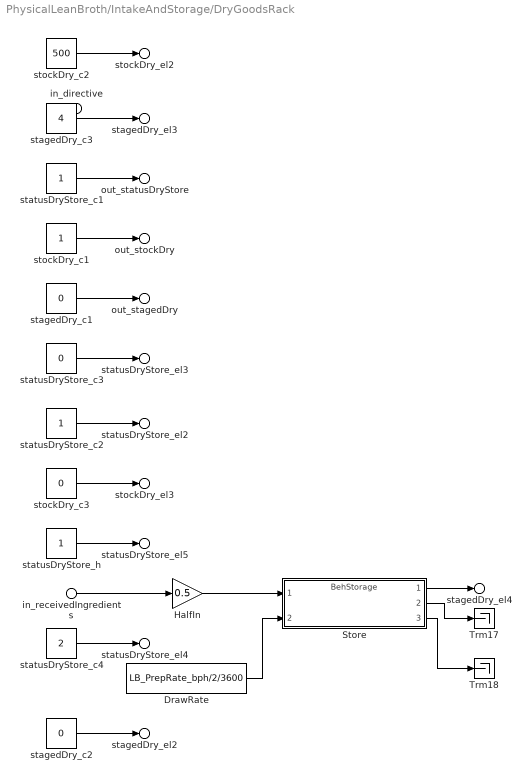
== system PhysicalLeanBroth/IntakeAndStorage/DryGoodsRack ==
  in_receivedIngredients : Inport  PortName=receivedIngredients  Element=flow_bps
  in_directive : Inport  Port=2  PortName=directive  Element=setpoint
  DrawRate : Constant  Value=LB_PrepRate_bph/2/3600
  HalfIn : Gain  Gain=0.5
  Store : ModelReference  ModelNameDialog=BehStorage  UsingDefaultArgumentValue=0,0  SimulationMode=Normal  ModelReferenceVersion=1.4
  Trm17 : Terminator
  Trm18 : Terminator
  stagedDry_c1 : Constant  Value=0
  stagedDry_c2 : Constant  Value=0
  stagedDry_c3 : Constant  Value=4
  statusDryStore_c1 : Constant
  statusDryStore_c2 : Constant
  statusDryStore_c3 : Constant  Value=0
  statusDryStore_c4 : Constant  Value=2
  statusDryStore_h : Constant
  stockDry_c1 : Constant
  stockDry_c2 : Constant  Value=500
  stockDry_c3 : Constant  Value=0
  out_stagedDry : Outport  PortName=stagedDry  Element=palletId
  stagedDry_el2 : Outport  PortName=stagedDry  Element=mass_kg
  stagedDry_el3 : Outport  PortName=stagedDry  Element=temp_C
  stagedDry_el4 : Outport  PortName=stagedDry  Element=flow_bps
  out_stockDry : Outport  Port=2  PortName=stockDry  Element=itemId
  stockDry_el2 : Outport  Port=2  PortName=stockDry  Element=qty_units
  stockDry_el3 : Outport  Port=2  PortName=stockDry  Element=error_pct
  out_statusDryStore : Outport  Port=3  PortName=statusDryStore  Element=unitId
  statusDryStore_el2 : Outport  Port=3  PortName=statusDryStore  Element=opState
  statusDryStore_el3 : Outport  Port=3  PortName=statusDryStore  Element=faultCode
  statusDryStore_el4 : Outport  Port=3  PortName=statusDryStore  Element=power_kW
  statusDryStore_el5 : Outport  Port=3  PortName=statusDryStore  Element=health
  wires:
  statusDryStore_c1/1 -> out_statusDryStore/1
  statusDryStore_h/1 -> statusDryStore_el5/1
  stockDry_c2/1 -> stockDry_el2/1
  stagedDry_c3/1 -> stagedDry_el3/1
  stockDry_c1/1 -> out_stockDry/1
  stagedDry_c1/1 -> out_stagedDry/1
  statusDryStore_c3/1 -> statusDryStore_el3/1
  statusDryStore_c2/1 -> statusDryStore_el2/1
  stockDry_c3/1 -> stockDry_el3/1
  Store/2 -> Trm17/1
  in_receivedIngredients/1 -> HalfIn/1
  statusDryStore_c4/1 -> statusDryStore_el4/1
  stagedDry_c2/1 -> stagedDry_el2/1
  HalfIn/1 -> Store/1
  DrawRate/1 -> Store/2
  Store/1 -> stagedDry_el4/1
  Store/3 -> Trm18/1

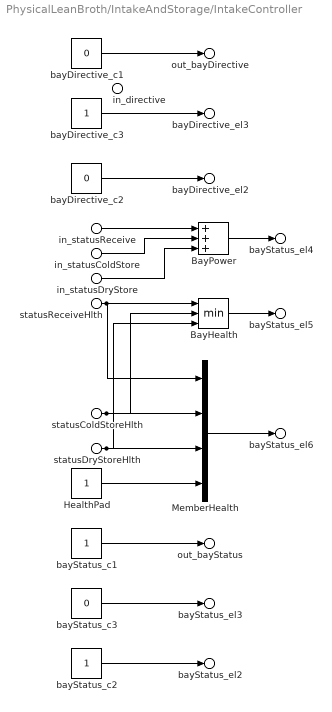
== system PhysicalLeanBroth/IntakeAndStorage/IntakeController ==
  in_directive : Inport  PortName=directive
  in_statusColdStore : Inport  Port=2  PortName=statusColdStore  Element=power_kW
  statusColdStoreHlth : Inport  Port=2  PortName=statusColdStore  Element=health
  in_statusDryStore : Inport  Port=3  PortName=statusDryStore  Element=power_kW
  statusDryStoreHlth : Inport  Port=3  PortName=statusDryStore  Element=health
  in_statusReceive : Inport  Port=4  PortName=statusReceive  Element=power_kW
  statusReceiveHlth : Inport  Port=4  PortName=statusReceive  Element=health
  BayHealth : MinMax  Inputs=3
  BayPower : Sum  Inputs=+++
  HealthPad : Constant
  MemberHealth : Mux
  bayDirective_c1 : Constant  Value=0
  bayDirective_c2 : Constant  Value=0
  bayDirective_c3 : Constant
  bayStatus_c1 : Constant
  bayStatus_c2 : Constant
  bayStatus_c3 : Constant  Value=0
  out_bayDirective : Outport  PortName=bayDirective  Element=cmdType
  bayDirective_el2 : Outport  PortName=bayDirective  Element=targetId
  bayDirective_el3 : Outport  PortName=bayDirective  Element=setpoint
  out_bayStatus : Outport  Port=2  PortName=bayStatus  Element=unitId
  bayStatus_el2 : Outport  Port=2  PortName=bayStatus  Element=opState
  bayStatus_el3 : Outport  Port=2  PortName=bayStatus  Element=faultCode
  bayStatus_el4 : Outport  Port=2  PortName=bayStatus  Element=power_kW
  bayStatus_el5 : Outport  Port=2  PortName=bayStatus  Element=health
  bayStatus_el6 : Outport  Port=2  PortName=bayStatus  Element=lineHealth
  wires:
  bayDirective_c1/1 -> out_bayDirective/1
  bayDirective_c3/1 -> bayDirective_el3/1
  bayDirective_c2/1 -> bayDirective_el2/1
  in_statusDryStore/1 -> BayPower/3
  in_statusReceive/1 -> BayPower/1
  in_statusColdStore/1 -> BayPower/2
  statusReceiveHlth/1 -> MemberHealth/1, BayHealth/1
  statusColdStoreHlth/1 -> BayHealth/2, MemberHealth/2
  bayStatus_c3/1 -> bayStatus_el3/1
  statusDryStoreHlth/1 -> BayHealth/3, MemberHealth/3
  HealthPad/1 -> MemberHealth/4
  bayStatus_c1/1 -> out_bayStatus/1
  bayStatus_c2/1 -> bayStatus_el2/1
  BayPower/1 -> bayStatus_el4/1
  BayHealth/1 -> bayStatus_el5/1
  MemberHealth/1 -> bayStatus_el6/1

== system PhysicalLeanBroth/IntakeAndStorage/ManualReceivingBay ==
  in_inboundCargo : Inport  PortName=inboundCargo  Element=flow_bps
  in_directive : Inport  Port=2  PortName=directive
  in_inboundCargoCap : Saturate  UpperLimit=0.0694444444444  LowerLimit=0
  receivedIngredients_c1 : Constant  Value=0
  receivedIngredients_c2 : Constant  Value=0
  receivedIngredients_c3 : Constant  Value=4
  statusReceive_c1 : Constant
  statusReceive_c2 : Constant
  statusReceive_c3 : Constant  Value=0
  statusReceive_c4 : Constant  Value=5
  statusReceive_h : Constant
  out_receivedIngredients : Outport  PortName=receivedIngredients  Element=palletId
  receivedIngredients_el2 : Outport  PortName=receivedIngredients  Element=mass_kg
  receivedIngredients_el3 : Outport  PortName=receivedIngredients  Element=temp_C
  receivedIngredients_el4 : Outport  PortName=receivedIngredients  Element=flow_bps
  out_statusReceive : Outport  Port=2  PortName=statusReceive  Element=unitId
  statusReceive_el2 : Outport  Port=2  PortName=statusReceive  Element=opState
  statusReceive_el3 : Outport  Port=2  PortName=statusReceive  Element=faultCode
  statusReceive_el4 : Outport  Port=2  PortName=statusReceive  Element=power_kW
  statusReceive_el5 : Outport  Port=2  PortName=statusReceive  Element=health
  wires:
  receivedIngredients_c1/1 -> out_receivedIngredients/1
  receivedIngredients_c3/1 -> receivedIngredients_el3/1
  statusReceive_h/1 -> statusReceive_el5/1
  statusReceive_c1/1 -> out_statusReceive/1
  statusReceive_c4/1 -> statusReceive_el4/1
  statusReceive_c2/1 -> statusReceive_el2/1
  receivedIngredients_c2/1 -> receivedIngredients_el2/1
  in_inboundCargo/1 -> in_inboundCargoCap/1
  statusReceive_c3/1 -> statusReceive_el3/1
  in_inboundCargoCap/1 -> receivedIngredients_el4/1

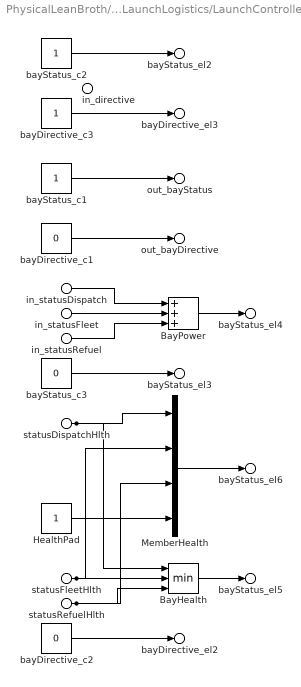
== system PhysicalLeanBroth/LaunchLogistics/LaunchController ==
  in_directive : Inport  PortName=directive
  in_statusRefuel : Inport  Port=2  PortName=statusRefuel  Element=power_kW
  statusRefuelHlth : Inport  Port=2  PortName=statusRefuel  Element=health
  in_statusDispatch : Inport  Port=3  PortName=statusDispatch  Element=power_kW
  statusDispatchHlth : Inport  Port=3  PortName=statusDispatch  Element=health
  in_statusFleet : Inport  Port=4  PortName=statusFleet  Element=power_kW
  statusFleetHlth : Inport  Port=4  PortName=statusFleet  Element=health
  BayHealth : MinMax  Inputs=3
  BayPower : Sum  Inputs=+++
  HealthPad : Constant
  MemberHealth : Mux
  bayDirective_c1 : Constant  Value=0
  bayDirective_c2 : Constant  Value=0
  bayDirective_c3 : Constant
  bayStatus_c1 : Constant
  bayStatus_c2 : Constant
  bayStatus_c3 : Constant  Value=0
  out_bayDirective : Outport  PortName=bayDirective  Element=cmdType
  bayDirective_el2 : Outport  PortName=bayDirective  Element=targetId
  bayDirective_el3 : Outport  PortName=bayDirective  Element=setpoint
  out_bayStatus : Outport  Port=2  PortName=bayStatus  Element=unitId
  bayStatus_el2 : Outport  Port=2  PortName=bayStatus  Element=opState
  bayStatus_el3 : Outport  Port=2  PortName=bayStatus  Element=faultCode
  bayStatus_el4 : Outport  Port=2  PortName=bayStatus  Element=power_kW
  bayStatus_el5 : Outport  Port=2  PortName=bayStatus  Element=health
  bayStatus_el6 : Outport  Port=2  PortName=bayStatus  Element=lineHealth
  wires:
  bayStatus_c2/1 -> bayStatus_el2/1
  bayDirective_c3/1 -> bayDirective_el3/1
  bayStatus_c1/1 -> out_bayStatus/1
  bayDirective_c1/1 -> out_bayDirective/1
  in_statusDispatch/1 -> BayPower/1
  bayStatus_c3/1 -> bayStatus_el3/1
  in_statusRefuel/1 -> BayPower/3
  in_statusFleet/1 -> BayPower/2
  statusDispatchHlth/1 -> BayHealth/1, MemberHealth/1
  HealthPad/1 -> MemberHealth/4
  statusFleetHlth/1 -> MemberHealth/2, BayHealth/2
  statusRefuelHlth/1 -> MemberHealth/3, BayHealth/3
  bayDirective_c2/1 -> bayDirective_el2/1
  BayPower/1 -> bayStatus_el4/1
  MemberHealth/1 -> bayStatus_el6/1
  BayHealth/1 -> bayStatus_el5/1

== system PhysicalLeanBroth/LaunchLogistics/RefuelSkid ==
  in_directive : Inport  PortName=directive
  statusRefuel_c1 : Constant
  statusRefuel_c2 : Constant
  statusRefuel_c3 : Constant  Value=0
  statusRefuel_c4 : Constant  Value=8
  statusRefuel_h : Constant
  out_statusRefuel : Outport  PortName=statusRefuel  Element=unitId
  statusRefuel_el2 : Outport  PortName=statusRefuel  Element=opState
  statusRefuel_el3 : Outport  PortName=statusRefuel  Element=faultCode
  statusRefuel_el4 : Outport  PortName=statusRefuel  Element=power_kW
  statusRefuel_el5 : Outport  PortName=statusRefuel  Element=health
  wires:
  statusRefuel_h/1 -> statusRefuel_el5/1
  statusRefuel_c3/1 -> statusRefuel_el3/1
  statusRefuel_c1/1 -> out_statusRefuel/1
  statusRefuel_c4/1 -> statusRefuel_el4/1
  statusRefuel_c2/1 -> statusRefuel_el2/1

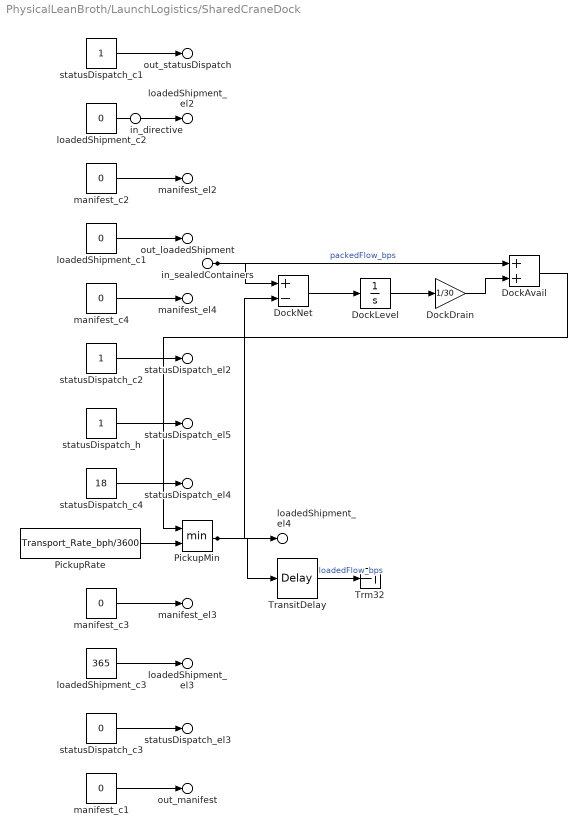
== system PhysicalLeanBroth/LaunchLogistics/SharedCraneDock ==
  in_sealedContainers : Inport  PortName=sealedContainers  Element=flow_bps
  in_directive : Inport  Port=2  PortName=directive
  DockAvail : Sum
  DockDrain : Gain  Gain=1/30
  DockLevel : Integrator  LimitOutput=on  UpperSaturationLimit=600  LowerSaturationLimit=0
  DockNet : Sum  Inputs=+-
  PickupMin : MinMax  Inputs=2
  PickupRate : Constant  Value=Transport_Rate_bph/3600
  TransitDelay : TransportDelay  DelayTime=Transport_Latency_s
  Trm32 : Terminator
  loadedShipment_c1 : Constant  Value=0
  loadedShipment_c2 : Constant  Value=0
  loadedShipment_c3 : Constant  Value=365
  manifest_c{1..4} (4 alike) : Constant  Value=0
  statusDispatch_c1 : Constant
  statusDispatch_c2 : Constant
  statusDispatch_c3 : Constant  Value=0
  statusDispatch_c4 : Constant  Value=18
  statusDispatch_h : Constant
  out_loadedShipment : Outport  PortName=loadedShipment  Element=batchId
  loadedShipment_el2 : Outport  PortName=loadedShipment  Element=count
  loadedShipment_el3 : Outport  PortName=loadedShipment  Element=sealRating_days
  loadedShipment_el4 : Outport  PortName=loadedShipment  Element=flow_bps
  out_manifest : Outport  Port=2  PortName=manifest  Element=destinationId
  manifest_el2 : Outport  Port=2  PortName=manifest  Element=batchId
  manifest_el3 : Outport  Port=2  PortName=manifest  Element=count
  manifest_el4 : Outport  Port=2  PortName=manifest  Element=mass_kg
  out_statusDispatch : Outport  Port=3  PortName=statusDispatch  Element=unitId
  statusDispatch_el2 : Outport  Port=3  PortName=statusDispatch  Element=opState
  statusDispatch_el3 : Outport  Port=3  PortName=statusDispatch  Element=faultCode
  statusDispatch_el4 : Outport  Port=3  PortName=statusDispatch  Element=power_kW
  statusDispatch_el5 : Outport  Port=3  PortName=statusDispatch  Element=health
  wires:
  statusDispatch_h/1 -> statusDispatch_el5/1
  statusDispatch_c1/1 -> out_statusDispatch/1
  DockNet/1 -> DockLevel/1
  loadedShipment_c2/1 -> loadedShipment_el2/1
  statusDispatch_c2/1 -> statusDispatch_el2/1
  manifest_c2/1 -> manifest_el2/1
  loadedShipment_c1/1 -> out_loadedShipment/1
  statusDispatch_c4/1 -> statusDispatch_el4/1
  manifest_c4/1 -> manifest_el4/1
  PickupRate/1 -> PickupMin/2
  manifest_c1/1 -> out_manifest/1
  manifest_c3/1 -> manifest_el3/1
  loadedShipment_c3/1 -> loadedShipment_el3/1
  statusDispatch_c3/1 -> statusDispatch_el3/1
  in_sealedContainers/1 -> DockAvail/1, DockNet/1  "packedFlow_bps"
  PickupMin/1 -> DockNet/2, loadedShipment_el4/1, TransitDelay/1
  TransitDelay/1 -> Trm32/1  "loadedFlow_bps"
  DockLevel/1 -> DockDrain/1
  DockDrain/1 -> DockAvail/2
  DockAvail/1 -> PickupMin/1

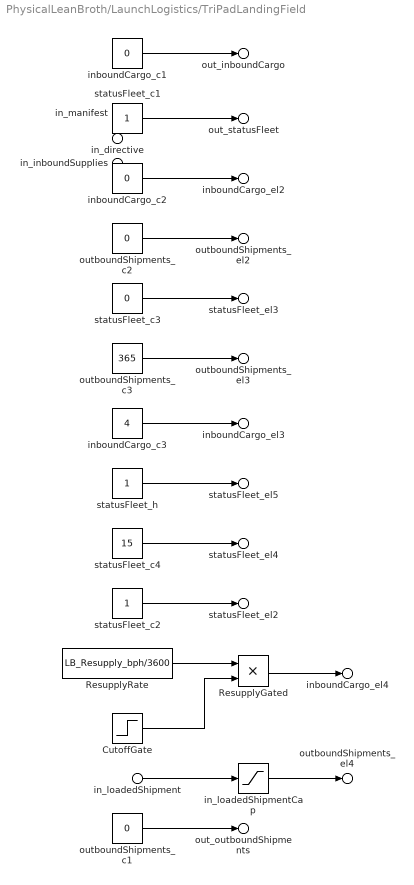
== system PhysicalLeanBroth/LaunchLogistics/TriPadLandingField ==
  in_loadedShipment : Inport  PortName=loadedShipment  Element=flow_bps
  in_manifest : Inport  Port=2  PortName=manifest
  in_directive : Inport  Port=3  PortName=directive
  in_inboundSupplies : Inport  Port=4  PortName=inboundSupplies
  CutoffGate : Step  Time=Resupply_Cutoff_T  InitialValue=1  FinalValue=0  SampleTime=0
  ResupplyGated : Product
  ResupplyRate : Constant  Value=LB_Resupply_bph/3600
  in_loadedShipmentCap : Saturate  UpperLimit=0.0666666666667  LowerLimit=0
  inboundCargo_c1 : Constant  Value=0
  inboundCargo_c2 : Constant  Value=0
  inboundCargo_c3 : Constant  Value=4
  outboundShipments_c1 : Constant  Value=0
  outboundShipments_c2 : Constant  Value=0
  outboundShipments_c3 : Constant  Value=365
  statusFleet_c1 : Constant
  statusFleet_c2 : Constant
  statusFleet_c3 : Constant  Value=0
  statusFleet_c4 : Constant  Value=15
  statusFleet_h : Constant
  out_inboundCargo : Outport  PortName=inboundCargo  Element=palletId
  inboundCargo_el2 : Outport  PortName=inboundCargo  Element=mass_kg
  inboundCargo_el3 : Outport  PortName=inboundCargo  Element=temp_C
  inboundCargo_el4 : Outport  PortName=inboundCargo  Element=flow_bps
  out_outboundShipments : Outport  Port=2  PortName=outboundShipments  Element=batchId
  outboundShipments_el2 : Outport  Port=2  PortName=outboundShipments  Element=count
  outboundShipments_el3 : Outport  Port=2  PortName=outboundShipments  Element=sealRating_days
  outboundShipments_el4 : Outport  Port=2  PortName=outboundShipments  Element=flow_bps
  out_statusFleet : Outport  Port=3  PortName=statusFleet  Element=unitId
  statusFleet_el2 : Outport  Port=3  PortName=statusFleet  Element=opState
  statusFleet_el3 : Outport  Port=3  PortName=statusFleet  Element=faultCode
  statusFleet_el4 : Outport  Port=3  PortName=statusFleet  Element=power_kW
  statusFleet_el5 : Outport  Port=3  PortName=statusFleet  Element=health
  wires:
  outboundShipments_c3/1 -> outboundShipments_el3/1
  inboundCargo_c1/1 -> out_inboundCargo/1
  statusFleet_h/1 -> statusFleet_el5/1
  statusFleet_c1/1 -> out_statusFleet/1
  outboundShipments_c2/1 -> outboundShipments_el2/1
  inboundCargo_c2/1 -> inboundCargo_el2/1
  statusFleet_c3/1 -> statusFleet_el3/1
  inboundCargo_c3/1 -> inboundCargo_el3/1
  statusFleet_c4/1 -> statusFleet_el4/1
  statusFleet_c2/1 -> statusFleet_el2/1
  ResupplyRate/1 -> ResupplyGated/1
  CutoffGate/1 -> ResupplyGated/2
  in_loadedShipment/1 -> in_loadedShipmentCap/1
  outboundShipments_c1/1 -> out_outboundShipments/1
  ResupplyGated/1 -> inboundCargo_el4/1
  in_loadedShipmentCap/1 -> outboundShipments_el4/1

== system PhysicalLeanBroth/PlantServices/AGVCartPool ==
  in_transportDirective : Inport  PortName=transportDirective
  statusTransport_c1 : Constant
  statusTransport_c2 : Constant
  statusTransport_c3 : Constant  Value=0
  statusTransport_c4 : Constant  Value=8
  statusTransport_h : Constant
  out_statusTransport : Outport  PortName=statusTransport  Element=unitId
  statusTransport_el2 : Outport  PortName=statusTransport  Element=opState
  statusTransport_el3 : Outport  PortName=statusTransport  Element=faultCode
  statusTransport_el4 : Outport  PortName=statusTransport  Element=power_kW
  statusTransport_el5 : Outport  PortName=statusTransport  Element=health
  wires:
  statusTransport_h/1 -> statusTransport_el5/1
  statusTransport_c3/1 -> statusTransport_el3/1
  statusTransport_c1/1 -> out_statusTransport/1
  statusTransport_c4/1 -> statusTransport_el4/1
  statusTransport_c2/1 -> statusTransport_el2/1

== system PhysicalLeanBroth/PlantServices/CompactFissionReactor ==
  in_directive : Inport  PortName=directive
  statusPower_c1 : Constant
  statusPower_c2 : Constant
  statusPower_c3 : Constant  Value=0
  statusPower_c4 : Constant  Value=0
  statusPower_h : Constant
  out_statusPower : Outport  PortName=statusPower  Element=unitId
  statusPower_el2 : Outport  PortName=statusPower  Element=opState
  statusPower_el3 : Outport  PortName=statusPower  Element=faultCode
  statusPower_el4 : Outport  PortName=statusPower  Element=power_kW
  statusPower_el5 : Outport  PortName=statusPower  Element=health
  wires:
  statusPower_h/1 -> statusPower_el5/1
  statusPower_c3/1 -> statusPower_el3/1
  statusPower_c1/1 -> out_statusPower/1
  statusPower_c4/1 -> statusPower_el4/1
  statusPower_c2/1 -> statusPower_el2/1

== system PhysicalLeanBroth/PlantServices/GravityCompUnit ==
  in_ambientGravity : Inport  PortName=ambientGravity  Element=gravity_g
  envStatus_c1 : Constant  Value=100
  out_envStatus : Outport  PortName=envStatus  Element=gravity_g
  envStatus_el2 : Outport  PortName=envStatus  Element=compensation_pct
  wires:
  in_ambientGravity/1 -> out_envStatus/1  "ambientGravity"
  envStatus_c1/1 -> envStatus_el2/1
